simulink model "tdoa_sim_energy"  (R2025a)
settings: Solver=FixedStepDiscrete  StartTime=0.0  StopTime=1.0  FixedStep=2.0833e-05  RelTol=1e-3
values from neighbouring files (symbols this model uses):
  audio1_vec = 0.2 * pulse    [model.m]
  audio2_vec = 0.5 * circshift(pulse,7)    [model.m]
  audio3_vec = 0.7 * circshift(pulse,11)    [model.m]
  c = 343    [model.m]
  energy_th = 0.05    [model.m]
  frame_len = 4096    [model.m]
  fs = 48000    [model.m]
  mic_positions = [0 2 1; 0 0 1.5]    [model.m]
settings Model: Creator=DELL  LastModifiedBy=DELL

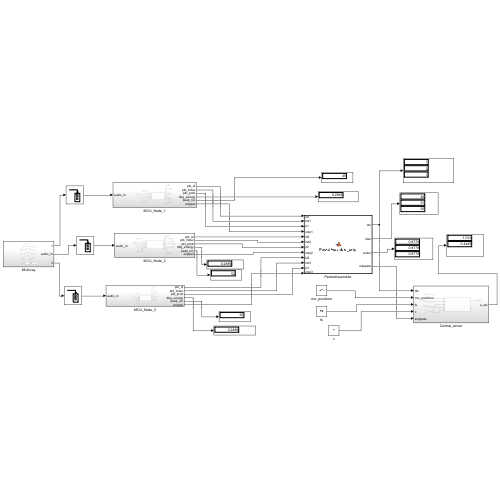
[thumbnail: Simulink's stored preview of the top-level diagram]
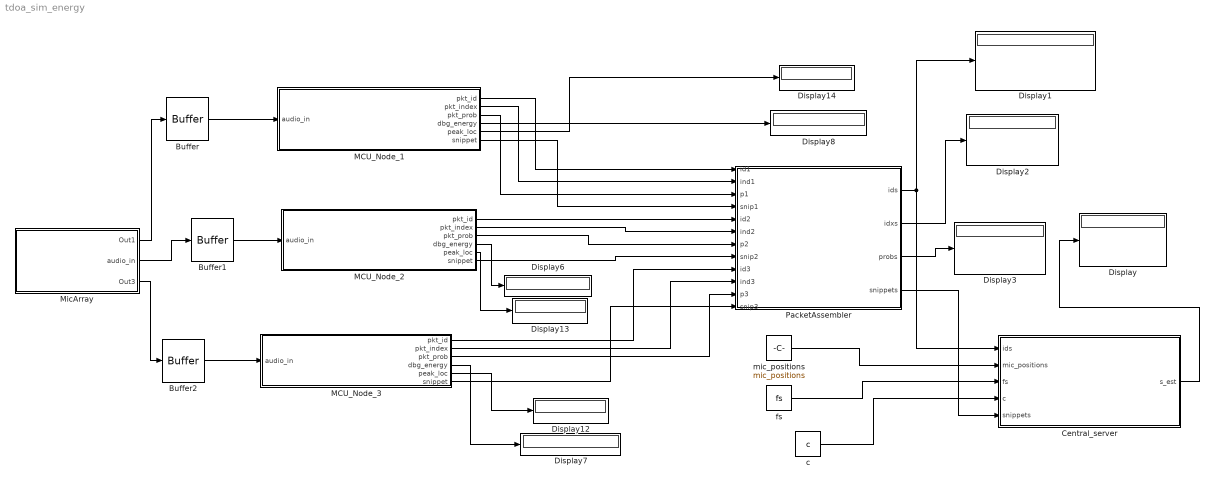
== system tdoa_sim_energy ==
  Buffer : Buffer  N=frame_len  OutputFrames=off
  Buffer1 : Buffer  N=frame_len  OutputFrames=off
  Buffer2 : Buffer  N=frame_len  OutputFrames=off
  Central_server : Subsystem
  Display{,1..3,6..8,12..14} (10 alike) : Display
  MCU_Node_1 : Subsystem
  MCU_Node_2 : Subsystem
  MCU_Node_3 : Subsystem
  MicArray : Subsystem
  PacketAssembler : MATLAB Function  TreatAsAtomicUnit=on
  c : Constant  Value=c
  fs : Constant  Value=fs
  mic_positions : Constant  Value=mic_positions
  wires:
  MicArray/1(Out1) -> Buffer/1
  MicArray/2(audio_in) -> Buffer1/1
  MicArray/3(Out3) -> Buffer2/1
  MCU_Node_1/1(pkt_id) -> PacketAssembler/1(id1)
  MCU_Node_1/2(pkt_index) -> PacketAssembler/2(ind1)
  MCU_Node_1/3(pkt_prob) -> PacketAssembler/3(p1)
  MCU_Node_2/1(pkt_id) -> PacketAssembler/5(id2)
  MCU_Node_2/2(pkt_index) -> PacketAssembler/6(ind2)
  MCU_Node_2/3(pkt_prob) -> PacketAssembler/7(p2)
  MCU_Node_3/1(pkt_id) -> PacketAssembler/9(id3)
  MCU_Node_3/2(pkt_index) -> PacketAssembler/10(ind3)
  MCU_Node_3/3(pkt_prob) -> PacketAssembler/11(p3)
  PacketAssembler/1(ids) -> Display1/1, Central_server/1(ids)
  PacketAssembler/2(idxs) -> Display2/1
  mic_positions/1 -> Central_server/2(mic_positions)
  c/1 -> Central_server/4(c)
  fs/1 -> Central_server/3(fs)
  Central_server/1(s_est) -> Display/1
  Buffer2/1 -> MCU_Node_3/1(audio_in)
  Buffer1/1 -> MCU_Node_2/1(audio_in)
  Buffer/1 -> MCU_Node_1/1(audio_in)
  MCU_Node_3/4(dbg_energy) -> Display7/1
  MCU_Node_2/4(dbg_energy) -> Display6/1
  MCU_Node_1/4(dbg_energy) -> Display8/1
  MCU_Node_2/5(peak_loc) -> Display13/1
  MCU_Node_1/5(peak_loc) -> Display14/1
  MCU_Node_3/5(peak_loc) -> Display12/1
  MCU_Node_1/6(snippet) -> PacketAssembler/4(snip1)
  MCU_Node_2/6(snippet) -> PacketAssembler/8(snip2)
  MCU_Node_3/6(snippet) -> PacketAssembler/12(snip3)
  PacketAssembler/4(snippets) -> Central_server/5(snippets)
  PacketAssembler/3(probs) -> Display3/1

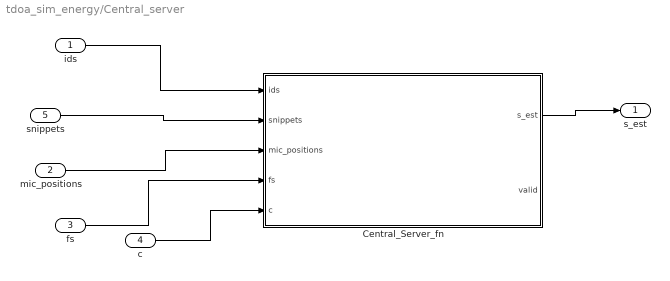
== system tdoa_sim_energy/Central_server ==
  ids : Inport
  mic_positions : Inport  Port=2
  fs : Inport  Port=3
  c : Inport  Port=4
  snippets : Inport  Port=5
  Central_Server_fn : MATLAB Function  TreatAsAtomicUnit=on
  s_est : Outport
  wires:
  Central_Server_fn/1(s_est) -> s_est/1
  ids/1 -> Central_Server_fn/1(ids)
  mic_positions/1 -> Central_Server_fn/3(mic_positions)
  fs/1 -> Central_Server_fn/4(fs)
  c/1 -> Central_Server_fn/5(c)
  snippets/1 -> Central_Server_fn/2(snippets)

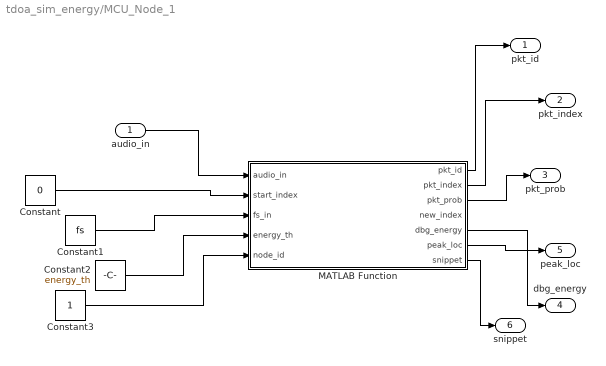
== system tdoa_sim_energy/MCU_Node_1 ==
  audio_in : Inport
  Constant : Constant  Value=0  SampleTime=-1
  Constant1 : Constant  Value=fs  SampleTime=-1
  Constant2 : Constant  Value=energy_th  SampleTime=-1
  Constant3 : Constant
  MATLAB Function : MATLAB Function  TreatAsAtomicUnit=on
  pkt_id : Outport
  pkt_index : Outport  Port=2
  pkt_prob : Outport  Port=3
  dbg_energy : Outport  Port=4
  peak_loc : Outport  Port=5
  snippet : Outport  Port=6
  wires:
  MATLAB Function/1(pkt_id) -> pkt_id/1
  MATLAB Function/2(pkt_index) -> pkt_index/1
  MATLAB Function/3(pkt_prob) -> pkt_prob/1
  Constant/1 -> MATLAB Function/2(start_index)
  audio_in/1 -> MATLAB Function/1(audio_in)
  Constant1/1 -> MATLAB Function/3(fs_in)
  Constant2/1 -> MATLAB Function/4(energy_th)
  Constant3/1 -> MATLAB Function/5(node_id)
  MATLAB Function/5(dbg_energy) -> dbg_energy/1
  MATLAB Function/6(peak_loc) -> peak_loc/1
  MATLAB Function/7(snippet) -> snippet/1

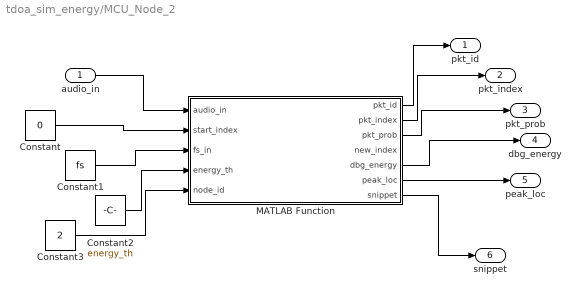
== system tdoa_sim_energy/MCU_Node_2 ==
  audio_in : Inport
  Constant : Constant  Value=0  SampleTime=-1
  Constant1 : Constant  Value=fs  SampleTime=-1
  Constant2 : Constant  Value=energy_th  SampleTime=-1
  Constant3 : Constant  Value=2
  MATLAB Function : MATLAB Function  TreatAsAtomicUnit=on
  pkt_id : Outport
  pkt_index : Outport  Port=2
  pkt_prob : Outport  Port=3
  dbg_energy : Outport  Port=4
  peak_loc : Outport  Port=5
  snippet : Outport  Port=6
  wires:
  MATLAB Function/3(pkt_prob) -> pkt_prob/1
  MATLAB Function/1(pkt_id) -> pkt_id/1
  MATLAB Function/2(pkt_index) -> pkt_index/1
  Constant1/1 -> MATLAB Function/3(fs_in)
  Constant2/1 -> MATLAB Function/4(energy_th)
  Constant3/1 -> MATLAB Function/5(node_id)
  audio_in/1 -> MATLAB Function/1(audio_in)
  Constant/1 -> MATLAB Function/2(start_index)
  MATLAB Function/5(dbg_energy) -> dbg_energy/1
  MATLAB Function/6(peak_loc) -> peak_loc/1
  MATLAB Function/7(snippet) -> snippet/1

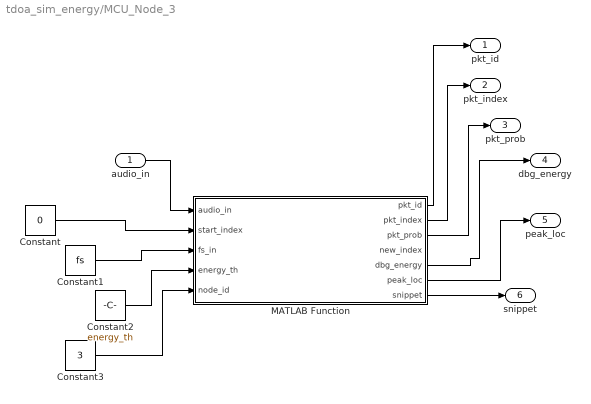
== system tdoa_sim_energy/MCU_Node_3 ==
  audio_in : Inport
  Constant : Constant  Value=0  SampleTime=-1
  Constant1 : Constant  Value=fs  SampleTime=-1
  Constant2 : Constant  Value=energy_th  SampleTime=-1
  Constant3 : Constant  Value=3
  MATLAB Function : MATLAB Function  TreatAsAtomicUnit=on
  pkt_id : Outport
  pkt_index : Outport  Port=2
  pkt_prob : Outport  Port=3
  dbg_energy : Outport  Port=4
  peak_loc : Outport  Port=5
  snippet : Outport  Port=6
  wires:
  MATLAB Function/3(pkt_prob) -> pkt_prob/1
  MATLAB Function/1(pkt_id) -> pkt_id/1
  MATLAB Function/2(pkt_index) -> pkt_index/1
  Constant3/1 -> MATLAB Function/5(node_id)
  Constant/1 -> MATLAB Function/2(start_index)
  Constant2/1 -> MATLAB Function/4(energy_th)
  audio_in/1 -> MATLAB Function/1(audio_in)
  Constant1/1 -> MATLAB Function/3(fs_in)
  MATLAB Function/5(dbg_energy) -> dbg_energy/1
  MATLAB Function/6(peak_loc) -> peak_loc/1
  MATLAB Function/7(snippet) -> snippet/1

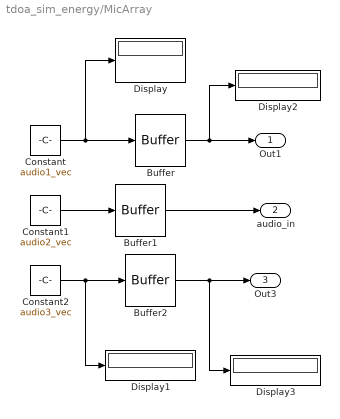
== system tdoa_sim_energy/MicArray ==
  Buffer : Buffer  N=frame_len  OutputFrames=off
  Buffer1 : Buffer  N=frame_len  OutputFrames=off
  Buffer2 : Buffer  N=frame_len  OutputFrames=off
  Constant : Constant  Value=audio1_vec  OutDataTypeStr=double
  Constant1 : Constant  Value=audio2_vec  OutDataTypeStr=double
  Constant2 : Constant  Value=audio3_vec  OutDataTypeStr=double
  Display{,1..3} (4 alike) : Display
  Out1 : Outport  VectorParamsAs1DForOutWhenUnconnected=off
  audio_in : Outport  Port=2  VectorParamsAs1DForOutWhenUnconnected=off
  Out3 : Outport  Port=3  VectorParamsAs1DForOutWhenUnconnected=off
  wires:
  Constant2/1 -> Display1/1, Buffer2/1
  Constant1/1 -> Buffer1/1
  Buffer2/1 -> Display3/1, Out3/1
  Buffer1/1 -> audio_in/1
  Buffer/1 -> Display2/1, Out1/1
  Constant/1 -> Display/1, Buffer/1

== matlab function tdoa_sim_energy/MCU_Node_2/MATLAB Function ==
  data: audio_in input double size=[frame_len 1]; pkt_id output double size=1; start_index input double size=1; fs_in input double size=1; pkt_index output double size=1; pkt_prob output double size=1; new_index output double size=1; energy_th input double size=1; node_id input double size=1; dbg_energy output double size=1; peak_loc output double size=1; snippet output double size=[512 1]
function [pkt_id, pkt_index, pkt_prob, new_index, dbg_energy, peak_loc, snippet] = MCU_Node_fn_snip( ...
    audio_in, start_index, fs_in, energy_th, node_id)
% Frame-based MCU node that detects an event and returns a fixed-length snippet
% FIXED snippet length L = 512 (compile-time constant)

%#codegen
L = 512;                % <--- FIXED compile-time constant, change here if desired

% default outputs
pkt_id = -1.0;
pkt_index = 0.0;
pkt_prob = 0.0;
dbg_energy = 0.0;
peak_loc = 0.0;

frame_len = double(length(audio_in));
new_index = double(start_index + frame_len);

% default snippet - fixed size
snippet = zeros(L,1);

% quantize / normalize (elementwise)
audio_q = round(audio_in .* (2^(15)-1)) ./ (2^(15)-1);

% compute energy and peak
dbg_energy = sum(audio_q .^ 2);
[~, local_peak] = max(abs(audio_q));   % 1..frame_len

% detection
if dbg_energy > energy_th
    pkt_id = double(node_id);
    pkt_index = double(start_index) + double(local_peak) - 1.0;
    peak_loc = double(local_peak);
    pkt_prob = min(1.0, (abs(audio_q(local_peak)) + dbg_energy) / (energy_th * 10.0));
    % extract snippet centered on local_peak into snippet(1:len)
    halfL = floor(L/2);
    s_idx = double(local_peak) - halfL;
    e_idx = s_idx + L - 1;
    % clamp indices
    if s_idx < 1
        s_idx = 1;
        e_idx = min(L, frame_len);
    end
    if e_idx > frame_len
        e_idx = frame_len;
        s_idx = max(1, frame_len - L + 1);
    end
    len = e_idx - s_idx + 1;
    snippet(1:len) = audio_in(s_idx:e_idx);
end
end

== matlab function tdoa_sim_energy/MCU_Node_1/MATLAB Function ==
  data: audio_in input double size=[frame_len 1]; pkt_id output double size=1; start_index input double size=1; fs_in input double size=1; pkt_index output double size=1; pkt_prob output double size=1; new_index output double size=1; energy_th input double size=1; node_id input double size=1; dbg_energy output double size=1; peak_loc output double size=1; snippet output double size=[512 1]
function [pkt_id, pkt_index, pkt_prob, new_index, dbg_energy, peak_loc, snippet] = MCU_Node_fn_snip( ...
    audio_in, start_index, fs_in, energy_th, node_id)
% Frame-based MCU node that detects an event and returns a fixed-length snippet
% FIXED snippet length L = 512 (compile-time constant)

%#codegen
L = 512;                % <--- FIXED compile-time constant, change here if desired

% default outputs
pkt_id = -1.0;
pkt_index = 0.0;
pkt_prob = 0.0;
dbg_energy = 0.0;
peak_loc = 0.0;

frame_len = double(length(audio_in));
new_index = double(start_index + frame_len);

% default snippet - fixed size
snippet = zeros(L,1);

% quantize / normalize (elementwise)
audio_q = round(audio_in .* (2^(15)-1)) ./ (2^(15)-1);

% compute energy and peak
dbg_energy = sum(audio_q .^ 2);
[~, local_peak] = max(abs(audio_q));   % 1..frame_len

% detection
if dbg_energy > energy_th
    pkt_id = double(node_id);
    pkt_index = double(start_index) + double(local_peak) - 1.0;
    peak_loc = double(local_peak);
    pkt_prob = min(1.0, (abs(audio_q(local_peak)) + dbg_energy) / (energy_th * 10.0));
    % extract snippet centered on local_peak into snippet(1:len)
    halfL = floor(L/2);
    s_idx = double(local_peak) - halfL;
    e_idx = s_idx + L - 1;
    % clamp indices
    if s_idx < 1
        s_idx = 1;
        e_idx = min(L, frame_len);
    end
    if e_idx > frame_len
        e_idx = frame_len;
        s_idx = max(1, frame_len - L + 1);
    end
    len = e_idx - s_idx + 1;
    snippet(1:len) = audio_in(s_idx:e_idx);
end
end

== matlab function tdoa_sim_energy/MCU_Node_3/MATLAB Function ==
  data: audio_in input double size=[frame_len 1]; pkt_id output double size=1; start_index input double size=1; fs_in input double size=1; pkt_index output double size=1; pkt_prob output double size=1; new_index output double size=1; energy_th input double size=1; node_id input double size=1; dbg_energy output double size=1; peak_loc output double size=1; snippet output double size=[512 1]
function [pkt_id, pkt_index, pkt_prob, new_index, dbg_energy, peak_loc, snippet] = MCU_Node_fn_snip( ...
    audio_in, start_index, fs_in, energy_th, node_id)
% Frame-based MCU node that detects an event and returns a fixed-length snippet
% FIXED snippet length L = 512 (compile-time constant)

%#codegen
L = 512;                % <--- FIXED compile-time constant, change here if desired

% default outputs
pkt_id = -1.0;
pkt_index = 0.0;
pkt_prob = 0.0;
dbg_energy = 0.0;
peak_loc = 0.0;

frame_len = double(length(audio_in));
new_index = double(start_index + frame_len);

% default snippet - fixed size
snippet = zeros(L,1);

% quantize / normalize (elementwise)
audio_q = round(audio_in .* (2^(15)-1)) ./ (2^(15)-1);

% compute energy and peak
dbg_energy = sum(audio_q .^ 2);
[~, local_peak] = max(abs(audio_q));   % 1..frame_len

% detection
if dbg_energy > energy_th
    pkt_id = double(node_id);
    pkt_index = double(start_index) + double(local_peak) - 1.0;
    peak_loc = double(local_peak);
    pkt_prob = min(1.0, (abs(audio_q(local_peak)) + dbg_energy) / (energy_th * 10.0));
    % extract snippet centered on local_peak into snippet(1:len)
    halfL = floor(L/2);
    s_idx = double(local_peak) - halfL;
    e_idx = s_idx + L - 1;
    % clamp indices
    if s_idx < 1
        s_idx = 1;
        e_idx = min(L, frame_len);
    end
    if e_idx > frame_len
        e_idx = frame_len;
        s_idx = max(1, frame_len - L + 1);
    end
    len = e_idx - s_idx + 1;
    snippet(1:len) = audio_in(s_idx:e_idx);
end
end

== matlab function tdoa_sim_energy/PacketAssembler ==
  data: id1 input; ids output; ind1 input; p1 input; snip1 input size=[snippet_len 1]; id2 input; ind2 input; p2 input; snip2 input size=[snippet_len 1]; id3 input; ind3 input; p3 input; idxs output; probs output size=[3 1]; snip3 input size=[snippet_len 1]; snippets output size=[snippet_len 3]
function [ids, idxs, probs, snippets] = PacketAssembler_snip( ...
    id1, ind1, p1, snip1, id2, ind2, p2, snip2, id3, ind3, p3, snip3)
%#codegen
% Assemble outputs from 3 MCU nodes into arrays and a snippets matrix
% Inputs:
%   idX, indX, pX  : scalars
%   snipX          : [L x 1] vector
% Outputs:
%   ids   : [3 x 1]
%   idxs  : [3 x 1]
%   probs  : [3 x 1]
%   snippets : [L x 3]  (columns are snip1, snip2, snip3)

% Assumes snip1/2/3 are same length L
L = size(snip1,1);

ids = [id1; id2; id3];
idxs = [ind1; ind2; ind3];
probs = [p1; p2; p3];

% pre-allocate snippets matrix and fill columns
snippets = zeros(L,3);
snippets(:,1) = snip1;
snippets(:,2) = snip2;
snippets(:,3) = snip3;

end

== matlab function tdoa_sim_energy/Central_server/Central_Server_fn ==
  data: ids input; s_est output; snippets input; mic_positions input; fs input; c input; valid output
function [s_est, valid] = Central_Server_fn(ids, snippets, mic_positions, fs, c)
% Central_Server_fn - GCC-PHAT based TDOA localization
% Inputs:
%   ids          : [N x 1] node ids (double)
%   snippets     : [L x N] snippet columns, each column is snippet from mic j
%   mic_positions: [2 x N] mic coordinates (meters)
%   fs           : sampling rate (Hz)
%   c            : speed of sound (m/s)
% Outputs:
%   s_est        : [2 x 1] estimated source location (m)
%   valid        : logical/double true if estimate computed

%#codegen
valid = false;
s_est = zeros(2,1);

% basic checks
if isempty(ids) || isempty(snippets) || size(snippets,2) < 3
    return;
end

N = size(snippets,2);
L = size(snippets,1);

% choose reference mic as column 1
ref = 1;

% Pre-allocate tdoa (seconds) vector for pairs ref->j
tdoa_meas = zeros(N-1,1);
pair_idx = 0;

% FFT length for cross-correlation (next pow of 2 >= 2*L)
nfft = 2^nextpow2(2*L);

% compute GCC-PHAT between ref and each other mic
Xref = fft(snippets(:,ref), nfft);
for j = 1:N
    if j == ref, continue; end
    pair_idx = pair_idx + 1;
    Xj = fft(snippets(:,j), nfft);
    R = Xref .* conj(Xj);
    % PHAT weight
    R = R ./ (abs(R) + eps);
    cc = ifft(R);
    % cc is length nfft, find peak and refine by parabolic interpolation
    % shift cross-corr so lags: -nfft/2..nfft/2-1
    ccmag = abs(cc);
    [~, Imax] = max(ccmag);
    % convert to zero-based index
    k = Imax - 1;
    % handle wrapping: convert index to signed lag in samples
    if k <= nfft/2 - 1
        lag = k;
    else
        lag = k - nfft;
    end
    % parabolic interpolation around Imax (use modular indexing)
    left = mod(Imax-2, nfft) + 1;
    right = mod(Imax, nfft) + 1;
    y1 = ccmag(left); y2 = ccmag(Imax); y3 = ccmag(right);
    denom = (y1 - 2*y2 + y3);
    if abs(denom) < eps
        delta = 0.0;
    else
        delta = 0.5 * (y1 - y3) / denom;   % fractional offset (samples)
    end
    lag_corrected = double(lag) + double(delta);
    % convert lag (samples) to time (seconds) t_ref - t_j
    tdoa_meas(pair_idx) = -lag_corrected / double(fs); 
    % NOTE: we used lag as index of cc = correlation ref vs j, and defined tdoa as (t_j - t_ref).
    % sign convention chosen so (di - dj)/c = tdoa_ref_j, solver below expects (di-dj)/c = tvec(i)-tvec(j)
end

% Build pairs array for solver: we will create pairs between mics [1..N] using ref as anchor
% Convert tdoa_meas to pairwise format consistent with solver: for i=ref and j others:
pairs = zeros(N-1,2);
for k = 1:(N-1)
    pairs(k,1) = ref;
    pairs(k,2) = k+1;
end

% initial guess: centroid of microphone positions
s = mean(mic_positions,2);

% Gauss-Newton solve (use same residual model as earlier)
for iter = 1:10
    m = size(pairs,1);
    r = zeros(m,1); J = zeros(m,2);
    for k = 1:m
        i = pairs(k,1);
        j = pairs(k,2);
        pi = mic_positions(:,i);
        pj = mic_positions(:,j);
        di = norm(s - pi); dj = norm(s - pj);
        if di == 0, di = 1e-6; end
        if dj == 0, dj = 1e-6; end
        % predicted TDOA (seconds) = (di - dj) / c
        pred = (di - dj) / c;
        r(k) = pred - tdoa_meas(k);
        J(k,1) = ((s(1)-pi(1))/di - (s(1)-pj(1))/dj) / c;
        J(k,2) = ((s(2)-pi(2))/di - (s(2)-pj(2))/dj) / c;
    end
    H = J' * J + 1e-6 * eye(2);
    delta = H \ (J' * r);
    s = s - delta;
    if norm(delta) < 1e-6
        break;
    end
end

s_est = s;
valid = true;
end
